simulink model "verify_UnglazedAbsorberISO2node_mdl"  (R2018b)
settings: Solver=ode45  StartTime=0.0  StopTime=14*3600  MaxStep=600  RelTol=1e-3  EnableMultiTasking=on
libraries: carnot x6, simulink x1
settings Model: Creator=drhf  LastModifiedBy=drhf
settings DataIOCC: SaveFormat=Array
settings OptimizationCC: ExpressionDepthLimit=2147483647  LifeSpan=inf
settings DebuggingCC: AlgebraicLoopMsg=none  UnderspecifiedInitializationDetection=Classic  MergeDetectMultiDrivingBlocksExec=none  SolverPrmCheckMsg=warning  StateNameClashWarn=warning  SFUnexpectedBacktrackingDiag=warning  SFNoUnconditionalDefaultTransitionDiag=warning  SFExecutionAtInitializationDiag=none
settings HardwareCC: ProdBitPerPointer=32  ProdBitPerSizeT=32  ProdBitPerPtrDiffT=32  ProdLargestAtomicFloat=None  ProdIntDivRoundTo=Undefined  ProdEndianess=Unspecified  ProdWordSize=32  ProdHWDeviceType=32-bit Generic
settings ModelReferenceCC: PropagateSignalLabelsOutOfModel=off
settings SFSimCC: SimUseLocalCustomCode=off
settings RTWCC: RTWUseLocalCustomCode=off
settings CodeAppCC: StateflowObjectComments=on
settings GRTTargetCC: TargetLangStandard=C89/C90 (ANSI)  GeneratePreprocessorConditionals=Disable all  CombineOutputUpdateFcns=off  GRTInterface=on
settings ConfigComp: CovMetricSettings=dw  CovHtmlReporting=on  CovSaveCumulativeToWorkspaceVar=on  CovSaveSingleToWorkspaceVar=on  CovExternalEMLEnable=off

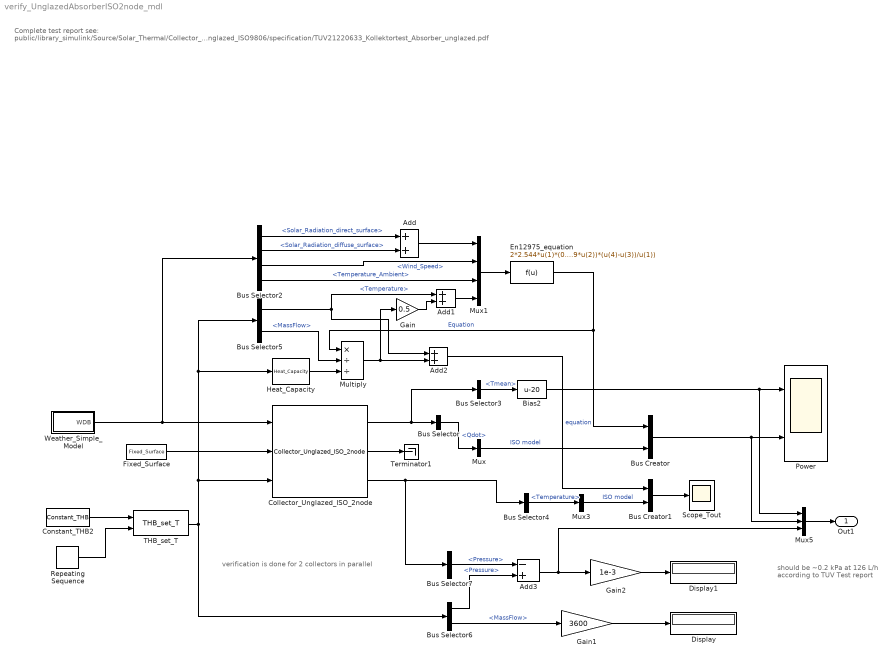
== system verify_UnglazedAbsorberISO2node_mdl ==
  note: verification is done for 2 collectors in parallel
  note: Complete test report see:
      | public/library_simulink/Source/Solar_Thermal/Collector_Unglazed_ISO9806/specification/TUV21220633_Kollektortest_Absorber_unglazed.pdf
  note: should be ~0.2 kPa at 126 L/h
      | according to TUV Test report
  Add : Sum  Inputs=2
  Add1 : Sum  Inputs=2
  Add2 : Sum  Inputs=2
  Add3 : Sum  Inputs=-+
  Bias2 : Bias  Bias=-20
  Bus Creator : BusCreator  Inputs=2
  Bus Creator1 : BusCreator  Inputs=2
  Bus Selector : BusSelector  OutputSignals=Qdot
  Bus Selector2 : BusSelector  OutputSignals=Solar_Radiation_direct_surface,Solar_Radiation_diffuse_surface,Wind_Speed,Temperature_Ambient
  Bus Selector3 : BusSelector  OutputSignals=Tmean
  Bus Selector4 : BusSelector  OutputSignals=Temperature
  Bus Selector5 : BusSelector  OutputSignals=Temperature,MassFlow
  Bus Selector6 : BusSelector  OutputSignals=Pressure,MassFlow
  Bus Selector7 : BusSelector  OutputSignals=Pressure
  Collector_Unglazed_ISO_2node : carnot/Source/Solar_Thermal/Collector_Unglazed_ISO_2node  tini=1  Ncollector=2  PathName='current'  FileName='Viessmann_SLK_ISO9806_lowCp.mat'  userPath=off  userParam=off  acol=2.544  len=2.1  eta0=0.702  bu=0.066  b1=32.64  b2=3.59  c_abs=2*3900  dplin=5504.4  dpqua=6222.096
      settings: SourceProductName=Carnot
  Constant_THB2 : carnot/Source/Simple/Constant_THB  t=10  mdot=2*126/3600  p=2e5  mID=No Pressure Drop  fluid=Water  mix=0  mix2=0  mix3=0  dia=0.02  hgt=0
      settings: SourceProductName=Carnot
  Display : Display
  Display1 : Display
  En12975_equation : Fcn  Expr=2*2.544*u(1)*(0.702*(1-0.066*u(2)) - (32.64 + 3.59*u(2))*(u(4)-u(3))/u(1))
  Fixed_Surface : carnot/Weather/Fixed_Surface  colangle=0  colazi=0  colrot=0
      settings: SourceProductName=Carnot
  Gain : Gain  Gain=0.5
  Gain1 : Gain  Gain=3600
  Gain2 : Gain  Gain=1e-3
  Heat_Capacity : carnot/Basic/Material_Properties/Heat_Capacity  VariantControl=CarlibClassic  INPUTARGUMENTS=THB  DEBUGLEVEL=DEBUGLEVEL  MAXTOTALWARNINGS=inf  MAXCONSECUTIVEWARNINGS=inf  WRITETOFILE=0  FILENAME='errors.txt'
      settings: SourceProductName=Carnot
  Multiply : Product  Inputs=*//
  Mux : Mux  Inputs=1
  Mux1 : Mux
  Mux3 : Mux  Inputs=1
  Mux5 : Mux  Inputs=3
  Power : Scope  NumInputPorts=2
  Repeating Sequence : simulink/Sources/Repeating Sequence  rep_seq_t=[0 0.5 14 15]*3600  rep_seq_y=[0.001 0.001 45 45]
  Scope_Tout : Scope
  THB_set_T : carnot/Source/Simple/THB_set_T
      settings: SourceProductName=Carnot
  Terminator1 : Terminator
  Weather_Simple_Model : Subsystem  mask{lat=60, Ibn=850, Idg=150, tamb=20, deltaTsky=-6, rh=50, precip=10e-3/24/3600           % 10 mm in 24 h, cloud=0.125, p=1013e2, vw=2, wdir=270}
      mask prompts: lat "Latitude in degree (north positve)"; Ibn "Maximum beam radiation on normal surface in W/m²"; Idg "Maximum diffuse radiation on horizontal surface in W/m²"; tamb "Ambient temperature in °C"; deltaTsky "Offset for sky temperature in K (usually -6K)"; rh "Relative humidity in %"; precip "Rainfall (precipitation) in m/s"; cloud "Cloud index in (0..1)"; p "Air pressure in Pa"; vw "Wind speed in m/s"; wdir "Wind direction in ° (0° = North, 90° = East)"
      mask DialogControl ParameterTabVar0 Prompt: Geography
      mask DialogControl ParameterTabVar01 Prompt: Weather
  Out1 : Outport
  wires:
  Gain2/1 -> Display1/1
  Mux3/1 -> Bus Creator1/2  "ISO model"
  Multiply/1 -> Add2/2, Gain/1
  Bus Selector6/2 -> Gain1/1  "<MassFlow>"
  Bus Selector2/2 -> Add/2  "<Solar_Radiation_diffuse_surface>"
  Bus Selector2/4 -> Mux1/3  "<Temperature_Ambient>"
  THB_set_T/1 -> Collector_Unglazed_ISO_2node/3, Bus Selector5/1, Heat_Capacity/1, Bus Selector6/1
  Collector_Unglazed_ISO_2node/3 -> Bus Selector7/1, Bus Selector4/1
  Bias2/1 -> Power/1, Mux5/1
  Mux/1 -> Bus Creator/2  "ISO model"
  Add2/1 -> Bus Creator1/1  "equation"
  Bus Selector7/1 -> Add3/1  "<Pressure>"
  Repeating Sequence/1 -> THB_set_T/2
  Bus Selector6/1 -> Add3/2  "<Pressure>"
  Bus Creator1/1 -> Scope_Tout/1
  Heat_Capacity/1 -> Multiply/3
  Gain/1 -> Add1/2
  Bus Selector5/2 -> Multiply/2  "<MassFlow>"
  Weather_Simple_Model/1(WDB) -> Collector_Unglazed_ISO_2node/1, Bus Selector2/1
  Bus Selector/1 -> Mux/1  "<Qdot>"
  Gain1/1 -> Display/1
  Bus Selector5/1 -> Add2/1, Add1/1  "<Temperature>"
  Bus Selector2/1 -> Add/1  "<Solar_Radiation_direct_surface>"
  Bus Selector2/3 -> Mux1/2  "<Wind_Speed>"
  Fixed_Surface/1 -> Collector_Unglazed_ISO_2node/2
  Collector_Unglazed_ISO_2node/2 -> Terminator1/1
  En12975_equation/1 -> Multiply/1, Bus Creator/1  "Equation"
  Add3/1 -> Mux5/3, Gain2/1
  Bus Creator/1 -> Mux5/2, Power/2
  Collector_Unglazed_ISO_2node/1 -> Bus Selector/1, Bus Selector3/1
  Constant_THB2/1 -> THB_set_T/1
  Add/1 -> Mux1/1
  Mux1/1 -> En12975_equation/1
  Bus Selector3/1 -> Bias2/1  "<Tmean>"
  Add1/1 -> Mux1/4
  Bus Selector4/1 -> Mux3/1  "<Temperature>"
  Mux5/1 -> Out1/1

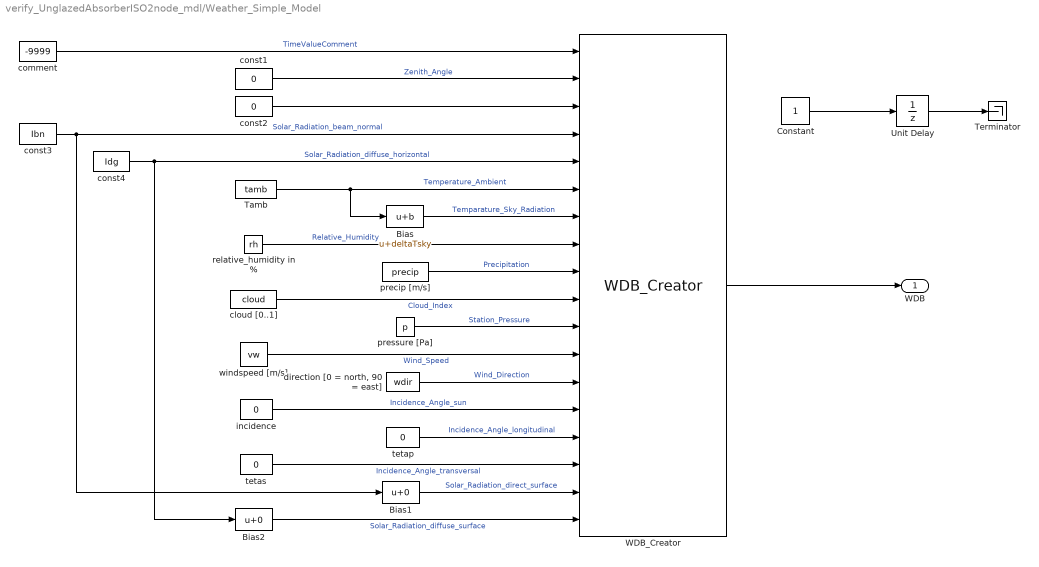
== system verify_UnglazedAbsorberISO2node_mdl/Weather_Simple_Model ==
  Bias : Bias  Bias=deltaTsky
  Bias1 : Bias
  Bias2 : Bias
  Constant : Constant
  Tamb : Constant  Value=tamb
  Terminator : Terminator
  Unit Delay : UnitDelay  SampleTime=3600
  WDB_Creator : carnot/Basic/Weather_and_Sun/WDB_Creator
      settings: SourceProductName=Carnot
  cloud [0..1] : Constant  Value=cloud
  comment : Constant  Value=-9999
  const1 : Constant  Value=0
  const2 : Constant  Value=0
  const3 : Constant  Value=Ibn
  const4 : Constant  Value=Idg
  "direction [0 = north, 90 = east]" : Constant  Value=wdir
  incidence : Constant  Value=0
  precip [m/s] : Constant  Value=precip
  pressure [Pa] : Constant  Value=p
  relative_humidity in % : Constant  Value=rh
  tetap : Constant  Value=0
  tetas : Constant  Value=0
  windspeed [m/s] : Constant  Value=vw
  WDB : Outport
  wires:
  WDB_Creator/1 -> WDB/1
  const3/1 -> Bias1/1, WDB_Creator/4  "Solar_Radiation_beam_normal"
  comment/1 -> WDB_Creator/1  "TimeValueComment"
  const1/1 -> WDB_Creator/2  "Zenith_Angle"
  const4/1 -> Bias2/1, WDB_Creator/5  "Solar_Radiation_diffuse_horizontal"
  Tamb/1 -> WDB_Creator/6, Bias/1  "Temperature_Ambient"
  Bias/1 -> WDB_Creator/7  "Temparature_Sky_Radiation"
  relative_humidity in %/1 -> WDB_Creator/8  "Relative_Humidity"
  precip [m/s]/1 -> WDB_Creator/9  "Precipitation"
  cloud [0..1]/1 -> WDB_Creator/10  "Cloud_Index"
  pressure [Pa]/1 -> WDB_Creator/11  "Station_Pressure"
  windspeed [m/s]/1 -> WDB_Creator/12  "Wind_Speed"
  "direction [0 = north, 90 = east]"/1 -> WDB_Creator/13  "Wind_Direction"
  incidence/1 -> WDB_Creator/14  "Incidence_Angle_sun"
  tetap/1 -> WDB_Creator/15  "Incidence_Angle_longitudinal"
  tetas/1 -> WDB_Creator/16  "Incidence_Angle_transversal"
  Bias1/1 -> WDB_Creator/17  "Solar_Radiation_direct_surface"
  Bias2/1 -> WDB_Creator/18  "Solar_Radiation_diffuse_surface"
  Constant/1 -> Unit Delay/1
  Unit Delay/1 -> Terminator/1
  const2/1 -> WDB_Creator/3
